simulink model "z1"  (R2017b)
settings: Solver=FixedStepDiscrete  StartTime=0.0  StopTime=0  RelTol=1e-3
undefined symbols (not defined in the file or in its folder): W
libraries: CPOiS_SourcesSinks x10, CPOiS_LinearTransforms x4, CPOiS_DataManipulation_DataTypeConversion x2
settings Model: Creator=alis  LastModifiedBy=alis

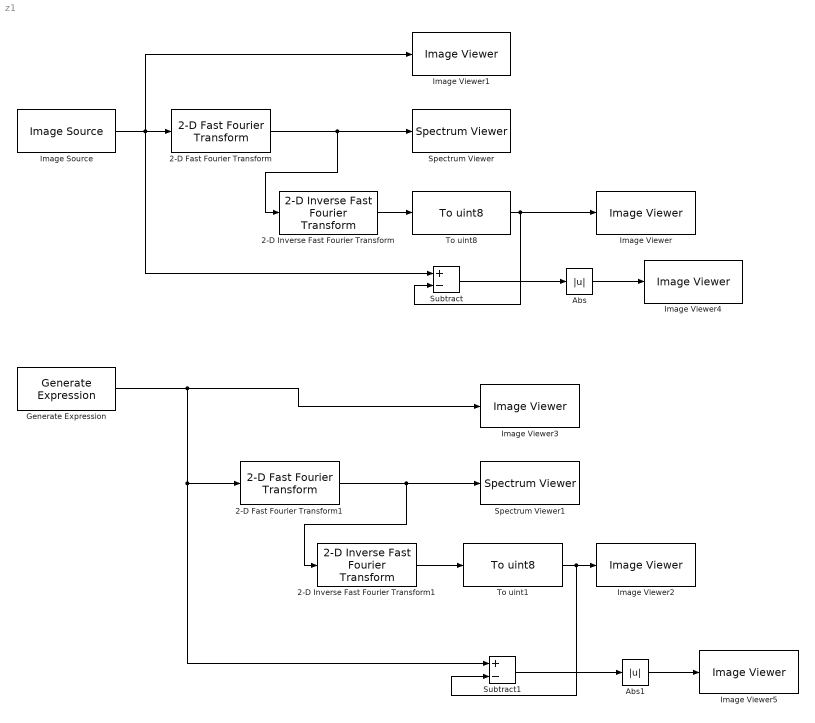
== system z1 ==
  2-D Fast Fourier Transform : CPOiS_LinearTransforms/2-D Fast Fourier Transform
      settings: SourceProductName=CPOiS - Digital image and signal processing
  2-D Fast Fourier Transform1 : CPOiS_LinearTransforms/2-D Fast Fourier Transform
      settings: SourceProductName=CPOiS - Digital image and signal processing
  2-D Inverse Fast Fourier Transform : CPOiS_LinearTransforms/2-D Inverse Fast  Fourier Transform
      settings: SourceProductName=CPOiS - Digital image and signal processing
  2-D Inverse Fast Fourier Transform1 : CPOiS_LinearTransforms/2-D Inverse Fast  Fourier Transform
      settings: SourceProductName=CPOiS - Digital image and signal processing
  Abs : Abs
  Abs1 : Abs
  Generate Expression : CPOiS_SourcesSinks/Generate Expression  Width=256  Height=256  Expression=128.*(sin(W)+1)
      settings: SourceProductName=CPOiS - Digital image and signal processing
  Image Source : CPOiS_SourcesSinks/Image Source  FileSelection=marine.png
      settings: SourceProductName=CPOiS - Digital image and signal processing
  Image Viewer{,1..5} (6 alike) : CPOiS_SourcesSinks/Image Viewer
      settings: SourceProductName=CPOiS - Digital image and signal processing
  Spectrum Viewer : CPOiS_SourcesSinks/Spectrum Viewer
      settings: SourceProductName=CPOiS - Digital image and signal processing
  Spectrum Viewer1 : CPOiS_SourcesSinks/Spectrum Viewer
      settings: SourceProductName=CPOiS - Digital image and signal processing
  Subtract : Sum  Inputs=+-
  Subtract1 : Sum  Inputs=+-
  To uint1 : CPOiS_DataManipulation_DataTypeConversion/To uint8
      settings: SourceProductName=CPOiS - Digital image and signal processing
  To uint8 : CPOiS_DataManipulation_DataTypeConversion/To uint8
      settings: SourceProductName=CPOiS - Digital image and signal processing
  wires:
  Image Source/1 -> Subtract/1, Image Viewer1/1, 2-D Fast Fourier Transform/1
  2-D Fast Fourier Transform/1 -> 2-D Inverse Fast Fourier Transform/1, Spectrum Viewer/1
  2-D Inverse Fast Fourier Transform/1 -> To uint8/1
  2-D Inverse Fast Fourier Transform1/1 -> To uint1/1
  2-D Fast Fourier Transform1/1 -> 2-D Inverse Fast Fourier Transform1/1, Spectrum Viewer1/1
  Generate Expression/1 -> Image Viewer3/1, Subtract1/1, 2-D Fast Fourier Transform1/1
  To uint8/1 -> Subtract/2, Image Viewer/1
  Subtract/1 -> Abs/1
  Abs/1 -> Image Viewer4/1
  Abs1/1 -> Image Viewer5/1
  To uint1/1 -> Subtract1/2, Image Viewer2/1
  Subtract1/1 -> Abs1/1
